simulink model "untitled"  (R2022a)
settings: Solver=VariableStepAuto  StartTime=0.0  StopTime=10  RelTol=1e-3
values from neighbouring files (symbols this model uses):
  C_PM = 1.758e-3    (= 0.001758)    [journal.m]
  Cfilter = 1/(Larm*wc2)    (= 4.78421193241e-05)    [journal.m]
  Cg = 50e-9    (= 5e-08)    [journal.m]
  Fc = Fnom*3.37    (= 168.5)    [journal.m]
  Fnom = 50    [journal.m]
  Inom = Pnom/(sqrt(3)*Vnom_dc)    [journal.m]
  Ki_Ireg = 6    [journal.m]
  Ki_Preg = 1.0    (= 1)    [journal.m]
  Ki_Qreg = 1.0    (= 1)    [journal.m]
  Ki_VDCreg = 100    [journal.m]
  Kp_Ireg = 0.6    [journal.m]
  Kp_Preg = 0.5/3    (= 0.166666666667)    [journal.m]
  Kp_Qreg = 0.5/3    (= 0.166666666667)    [journal.m]
  Kp_VDCreg = 4    [journal.m]
  L_cable = 15e-3    (= 0.015)    [journal.m]
  Larm = Larm_pu*(Zbase/(2*pi*Fnom))    (= 0.0529455974536)    [journal.m]
  Lff = Larm_pu/2    (= 0.075)    [journal.m]
  Lfilter = 0    [journal.m]
  Limits_Ireg = [ 2.0  -2.0]    [journal.m]
  Limits_Preg = [ 1.2, 0.8 ]    [journal.m]
  Limits_Qreg = [ 0.25, -0.25 ]    [journal.m]
  Limits_VDCreg = [ 2.0  -2.0]    [journal.m]
  Lxfo = 0.12    [journal.m]
  Nb_PM = 36    [journal.m]
  Pnom = 1000e6    (= 1000000000)    [journal.m]
  R_cable = 0.5    [journal.m]
  R_startup = 400    [journal.m]
  Rarm = Rarm_pu*Zbase    (= 0.1663335)    [journal.m]
  Rff = Rarm_pu/2    (= 0.00075)    [journal.m]
  Rfilter = 1/(Cfilter*w)*30    (= 1996.002)    [journal.m]
  Rg = 100    [journal.m]
  Rxfo = 0.003    [journal.m]
  Slope_Pref = 0.5    [journal.m]
  Slope_Qref = 0.5    [journal.m]
  Slope_Vdc_ref = Vnom_dc/5    (= 128000)    [journal.m]
  Tbrk1_On = 0.1    [journal.m]
  Tbrk2_On = 0.5    [journal.m]
  Tdeblock = 1    [journal.m]
  Tfault = 999    [journal.m]
  Ton_Converter2 = 2    [journal.m]
  Ton_PQreg = 2    [journal.m]
  Ton_VDCreg = 1    [journal.m]
  Ts = Ts_Control    (= 4e-05)    [journal.m]
  Ts_Control = 40e-6    (= 4e-05)    [journal.m]
  Ts_Power = 20e-6    (= 2e-05)    [journal.m]
  Vnom_dc = 640e3    (= 640000)    [journal.m]
  Vnom_prim = 400e3    (= 400000)    [journal.m]
  Vnom_sec = 333e3    (= 333000)    [journal.m]
undefined symbols (not defined in the file or in its folder): D11, Delta, DiscIntNeverNeededParam, find_system, Pcc, sigbuilder_block
libraries: powerlib_extras x42, spsSeriesRLCBranchLib x32, spsCurrentMeasurementLib x24, simulink x18, spsVoltageMeasurementLib x16, spsHalfBridgeMMCLib x12, spsThreePhaseVIMeasurementLib x10, simulink_extras x6, spsBreakerLib x6, spsParallelRLCBranchLib x6, spsThreePhaseBreakerLib x4, spsMeanLib x4
(part 2 of 6)

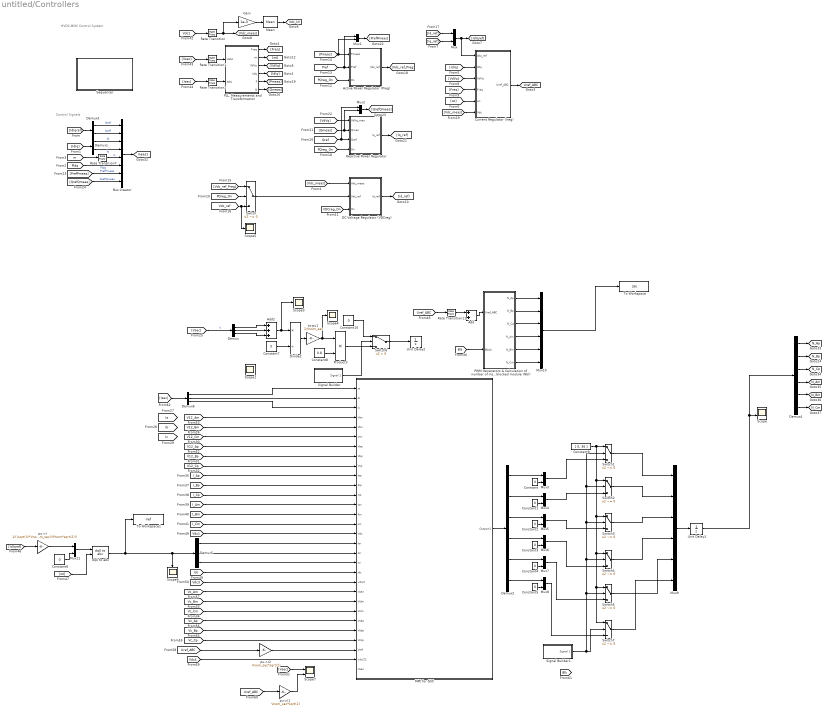
== system untitled/Controllers ==
  note: HVDC-MMC Control System
  note: Control Signals
  Active Power Regulator (Preg) : Subsystem
  Add : Sum
  Add2 : Sum  Inputs=+++
  Bus Creator : BusCreator  Inputs=8
  Constant{,1..6,10} (8 alike) : Constant  Value=0
  Constant7 : Constant  Value=3
  Constant8 : Constant  Value=0.8
  Constant9 : Constant  Value=[ 0, 36 ]
  Current Regulator (Ireg) : Subsystem
  DC Voltage Regulator (VDCreg) : Subsystem
  Demux : Demux  Outputs=3
  Demux1 : Demux  Outputs=2
  Demux2 : Demux  Outputs=6
  Demux3 : Demux  Outputs=2
  Demux4 : Demux  Outputs=6
  Demux5 : Demux  Outputs=3
  Demux6 : Demux  Outputs=3
  Divide2 : Product  Inputs=*/
  Gain : Gain  Gain=1e-3
  MPC for GSC : Subsystem
  Mean : spsMeanLib/Mean  Freq=Fnom/3  Vinit=0  Ts=Ts_Control
  Mux{,1..8,11} (10 alike) : Mux  Inputs=2
  Mux10 : Mux  Inputs=6
  Mux9 : Mux  Inputs=6
  "PLL, Measurements and Transformation" : Subsystem
  PWM Generators & Calculation of number of inserted modules (Nin) and number of blocked module (Nbl) : Subsystem
  Product3 : Product  RndMeth=Zero
  Rate Transition{,1..2,7} (4 alike) : RateTransition  OutPortSampleTime=Ts_Control
  Rate Transition11 : RateTransition  OutPortSampleTime=Ts_Power
  Reactive Power Regulator : Subsystem
  Scope : Scope  NumInputPorts=2
  Scope1 : Scope  NumInputPorts=2
  Scope{3..6} (4 alike) : Scope
  Scope7 : Scope  NumInputPorts=2
  Sequencer : Subsystem
      mask Display: disp('Sequencer')
  Signal Builder : Subsystem  Tag=STV Subsys  LoadFcn=sigbuilder_block('load');  StartFcn=sigbuilder_block('start');  StopFcn=sigbuilder_block('stop');  ClipboardFcn=sigbuilder_block('clipboard');  mask(Sigbuilder block){tuvar=[0:10]}
      mask help: Simulink:masks:SigbuilderBlock_MD
      mask init:
      | if ~strcmp(get_param(bdroot(gcbh),'SimulationStatus'),'stopped') tuvar = sigbuilder_block('maskInit'); end
      settings: CopyFcn=sigbuilder_block('copy');  DeleteFcn=sigbuilder_block('delete');  ModelCloseFcn=sigbuilder_block('modelClose');  PreSaveFcn=sigbuilder_block('preSave');  PauseFcn=sigbuilder_block('pause');  ContinueFcn=sigbuilder_block('continue');  NameChangeFcn=sigbuilder_block('namechange');  OpenFcn=sigbuilder_block('open',[0 36 1152 555.6 ]);  CloseFcn=sigbuilder_block('close');
      mask Display: plot(0, 0, 100, 100,[2, 2, 32, 32, 2], [68, 8, 8, 68, 68],[32, 2], [38, 38], [32, 19, 2],[53, 60, 44], [32, 17, 17, 2],[16, 16, 31, 31]);txt = getActiveGroup(gcbh);text(2, 100, txt,'verticalAlignment', 'top');
  Signal Builder1 : Subsystem  Tag=STV Subsys  LoadFcn=sigbuilder_block('load');  StartFcn=sigbuilder_block('start');  StopFcn=sigbuilder_block('stop');  ClipboardFcn=sigbuilder_block('clipboard');  mask(Sigbuilder block){tuvar=[0:10]}
      mask help: Simulink:masks:SigbuilderBlock_MD
      mask init:
      | if ~strcmp(get_param(bdroot(gcbh),'SimulationStatus'),'stopped') tuvar = sigbuilder_block('maskInit'); end
      settings: CopyFcn=sigbuilder_block('copy');  DeleteFcn=sigbuilder_block('delete');  ModelCloseFcn=sigbuilder_block('modelClose');  PreSaveFcn=sigbuilder_block('preSave');  PauseFcn=sigbuilder_block('pause');  ContinueFcn=sigbuilder_block('continue');  NameChangeFcn=sigbuilder_block('namechange');  OpenFcn=sigbuilder_block('open',[0 36 1152 555.6 ]);  CloseFcn=sigbuilder_block('close');
      mask Display: plot(0, 0, 100, 100,[2, 2, 32, 32, 2], [68, 8, 8, 68, 68],[32, 2], [38, 38], [32, 19, 2],[53, 60, 44], [32, 17, 17, 2],[16, 16, 31, 31]);txt = getActiveGroup(gcbh);text(2, 100, txt,'verticalAlignment', 'top');
  Switch{,1..5,7} (7 alike) : Switch  Criteria=u2 ~= 0  SaturateOnIntegerOverflow=off  InputSameDT=off
  Switch6 : Switch  Criteria=u2 > Threshold  SaturateOnIntegerOverflow=off  InputSameDT=off
  To Workspace : ToWorkspace  VariableName=SM  SaveFormat=Timeseries  SampleTime=-1
  To Workspace1 : ToWorkspace  VariableName=Iref  SaveFormat=Timeseries  SampleTime=-1
  Unit Delay1 : UnitDelay  SampleTime=-1
  Unit Delay2 : UnitDelay  SampleTime=-1
  dq0 to abc : spsdq0toabcLib/dq0 to abc  Alignment=90 degrees behind phase A axis
  pu->I : Gain  Gain=1/((sqrt(3)*Vnom_sec)/(Pnom*sqrt(2)))  SaturateOnIntegerOverflow=on  OutDataTypeStr=Inherit: Same as input  ParamDataTypeStr=Inherit: Same as input
  pu->I1 : Gain  Gain=Vnom_sec*sqrt(2)  SaturateOnIntegerOverflow=on  OutDataTypeStr=Inherit: Same as input  ParamDataTypeStr=Inherit: Same as input
  pu->I2 : Gain  Gain=Vnom_sec*sqrt(2)  SaturateOnIntegerOverflow=on  OutDataTypeStr=Inherit: Same as input  ParamDataTypeStr=Inherit: Same as input
  to-pu1 : Gain  Gain=1/Vnom_sec
  tag scope: N_Am=global, N_Ap=global, N_Bm=global, N_Bp=global, N_Cm=global, N_Cp=global, Uref_ABC=global, Vdc_kV=global, meas1=global
  wires:
  [Uref_ABC] -> Rate Transition11/1
  Mean/1 -> [Vdc_kV]
  [Vsec] -> Rate Transition1/1
  [Isec] -> Rate Transition2/1
  [Vdc_meas] -> Current Regulator (Ireg)/6(Vdc)
  [Vdc_meas] -> DC Voltage Regulator (VDCreg)/1(Vdc_meas)
  DC Voltage Regulator (VDCreg)/1(Id_ref) -> [Id_ref]
  Gain/1 -> Mean/1
  Current Regulator (Ireg)/1(Uref_ABC) -> [Uref_ABC]
  [wt] -> Current Regulator (Ireg)/5(wt)
  [Vdc1] -> Rate Transition/1
  "PLL, Measurements and Transformation"/2(wt) -> [wt]
  "PLL, Measurements and Transformation"/4(IdIq) -> [IdIq]
  [Freq] -> Current Regulator (Ireg)/4(Freq)
  [Id_ref] -> Mux/1
  "PLL, Measurements and Transformation"/3(VdVq) -> [VdVq]
  Mux/1 -> Current Regulator (Ireg)/1(IdIq_ref), [IdIqref]
  Demux1/2 -> Bus Creator/4  "Iq"
  [IdIq] -> Current Regulator (Ireg)/2(IdIq)
  [IdIqref] -> Demux3/1
  Demux3/1 -> Bus Creator/1  "Idref"
  [IdIq] -> Demux1/1
  Bus Creator/1 -> [meas1]
  Demux3/2 -> Bus Creator/2  "Iqref"
  [m] -> Rate Transition7/1
  Demux1/1 -> Bus Creator/3  "Id"
  [PIdq] -> Bus Creator/6  "PIdq"
  "PLL, Measurements and Transformation"/1(Freq) -> [Freq]
  [VdVq] -> Current Regulator (Ireg)/3(VdVq)
  [Iq_ref] -> Mux/2
  Rate Transition/1 -> Gain/1, [Vdc_meas]
  Rate Transition2/1 -> "PLL, Measurements and Transformation"/2(Iabc)
  Rate Transition7/1 -> Bus Creator/5  "m"
  Rate Transition1/1 -> "PLL, Measurements and Transformation"/1(Vabc)
  [Vdc_ref] -> Scope5/1, Switch/3
  [PQreg_On] -> Reactive Power Regulator/4(On)
  Mux2/1 -> [QrefQmeas]
  Mux1/1 -> [PrefPmeas]
  [Vdc_ref_Preg] -> Switch/1
  [Qref] -> Mux2/1, Reactive Power Regulator/3(Qref)
  [QrefQmeas] -> Bus Creator/8  "QrefQmeas"
  [VDCreg_On] -> DC Voltage Regulator (VDCreg)/3(On)
  [PQreg_On] -> Active Power Regulator (Preg)/3(On)
  Active Power Regulator (Preg)/1(Vdc_ref) -> [Vdc_ref_Preg]
  Reactive Power Regulator/1(Iq_ref) -> [Iq_ref]
  "PLL, Measurements and Transformation"/5(P) -> [Pmeas]
  [VdVq] -> Reactive Power Regulator/1(VdVq_mes)
  [Qmeas] -> Mux2/2, Reactive Power Regulator/2(Qmes)
  [PQreg_On] -> Switch/2
  Switch/1 -> DC Voltage Regulator (VDCreg)/2(Vdc_ref)
  [Pref] -> Active Power Regulator (Preg)/2(Pref), Mux1/1
  [PrefPmeas] -> Bus Creator/7  "PrefPmeas"
  "PLL, Measurements and Transformation"/6(Q) -> [Qmeas]
  [Pmeas] -> Active Power Regulator (Preg)/1(Pmeas), Mux1/2
  [Blk] -> PWM Generators & Calculation of number of inserted modules (Nin) and number of blocked module (Nbl)/2(Block)
  Demux/1 -> Add2/1
  Constant10/1 -> Switch6/1
  Constant7/1 -> Divide2/2
  to-pu1/1 -> Scope4/1, Product3/1
  Signal Builder/1(Signal 1) -> Switch6/2
  Demux/2 -> Add2/2
  Demux/3 -> Add2/3
  Add2/1 -> Scope3/1, Divide2/1
  Constant8/1 -> Product3/2
  Switch6/1 -> Unit Delay2/1
  Divide2/1 -> to-pu1/1
  [Vsec] -> Demux/1  "V"
  Rate Transition11/1 -> Add/1
  Add/1 -> PWM Generators & Calculation of number of inserted modules (Nin) and number of blocked module (Nbl)/1(Uref_ABC)
  Product3/1 -> Switch6/3
  PWM Generators & Calculation of number of inserted modules (Nin) and number of blocked module (Nbl)/1(N_Ap) -> Mux10/1
  PWM Generators & Calculation of number of inserted modules (Nin) and number of blocked module (Nbl)/2(N_Bp) -> Mux10/2
  PWM Generators & Calculation of number of inserted modules (Nin) and number of blocked module (Nbl)/3(N_Cp) -> Mux10/3
  PWM Generators & Calculation of number of inserted modules (Nin) and number of blocked module (Nbl)/4(N_Am) -> Mux10/4
  PWM Generators & Calculation of number of inserted modules (Nin) and number of blocked module (Nbl)/5(N_Bm) -> Mux10/5
  PWM Generators & Calculation of number of inserted modules (Nin) and number of blocked module (Nbl)/6(N_Cm) -> Mux10/6
  Demux4/1 -> [N_Ap]
  Demux4/2 -> [N_Bp]
  Demux4/3 -> [N_Cp]
  Demux4/4 -> [N_Am]
  Demux4/5 -> [N_Bm]
  Demux4/6 -> [N_Cm]
  [I_Bm] -> MPC for GSC/14(ibn)
  pu->I/1 -> Mux11/1
  [I_Ap] -> MPC for GSC/10(iap)
  [V12_Bp] -> MPC for GSC/8(Vbp)
  Mux11/1 -> dq0 to abc/1
  Demux2/4 -> Mux6/1
  Demux2/3 -> Mux5/1
  Demux2/5 -> Mux7/1
  Constant/1 -> Mux3/2
  [V12_Cp] -> MPC for GSC/9(Vcp)
  [V12_Bm] -> MPC for GSC/5(Vbn)
  [V12_Ap] -> MPC for GSC/7(Vap)
  Demux2/6 -> Mux8/1
  Constant1/1 -> Mux4/2
  [I_Am] -> MPC for GSC/13(ian)
  [Vdc1] -> MPC for GSC/16(Vdc)
  Demux6/2 -> MPC for GSC/2(ib)
  Demux5/2 -> MPC for GSC/18(ibr)
  Demux5/1 -> MPC for GSC/17(iar)
  Constant5/1 -> Mux8/2
  [wt] -> dq0 to abc/2
  Demux6/3 -> MPC for GSC/3(ic)
  Demux2/2 -> Mux4/1
  Constant4/1 -> Mux7/2
  [I_Bp] -> MPC for GSC/11(ibp)
  [IdIqref] -> pu->I/1
  [V12_Cm] -> MPC for GSC/6(Vcn)
  Constant6/1 -> Mux11/2
  Constant3/1 -> Mux6/2
  Demux5/3 -> MPC for GSC/19(icr)
  [V12_Am] -> MPC for GSC/4(Van)
  MPC for GSC/1(Outport1) -> Demux2/1
  Demux6/1 -> MPC for GSC/1(ia)
  [I_Cp] -> MPC for GSC/12(icp)
  [I_Cm] -> MPC for GSC/15(icn)
  Mux9/1 -> Unit Delay1/1
  Constant2/1 -> Mux5/2
  [Idc] -> MPC for GSC/20(idc)
  [Vdc3] -> MPC for GSC/21(vdc/2)
  [Vc_Am] -> MPC for GSC/22(Vcan)
  [Vc_Bm] -> MPC for GSC/23(Vcbn)
  [Vc_Cm] -> MPC for GSC/24(Vccn)
  [Vc_Ap] -> MPC for GSC/25(Vcap)
  [Vc_Bp] -> MPC for GSC/26(Vcbp)
  [Vc_Cp] -> MPC for GSC/27(Vccp)
  [Vdc4] -> MPC for GSC/29(vdc/21)
  [Uref_ABC] -> pu->I1/1
  Demux2/1 -> Mux3/1
  Mux10/1 -> To Workspace/1
  Mux7/1 -> Switch5/3
  Mux4/1 -> Switch2/3
  Mux6/1 -> Switch4/3
  Signal Builder1/1(Signal 1) -> Switch1/2, Switch2/2, Switch3/2, Switch4/2, Switch5/2, Switch7/2
  Mux8/1 -> Switch7/3
  Switch7/1 -> Mux9/6
  Switch4/1 -> Mux9/4
  Switch5/1 -> Mux9/5
  Mux3/1 -> Switch1/3
  Switch2/1 -> Mux9/2
  Mux5/1 -> Switch3/3
  Constant9/1 -> Switch1/1, Switch7/1, Switch5/1, Switch4/1, Switch3/1, Switch2/1
  Switch3/1 -> Mux9/3
  Switch1/1 -> Mux9/1
  pu->I1/1 -> Scope7/2
  ? -> MPC for GSC/30(Vsec)
  [Vsec] -> Scope7/1
  [Uref_ABC] -> pu->I2/1
  pu->I2/1 -> MPC for GSC/28(Vref)
  [Isec] -> Demux6/1
  Unit Delay1/1 -> Demux4/1, Scope/2
  ? -> Scope/1
  dq0 to abc/1 -> To Workspace1/1, Demux5/1, Scope6/1

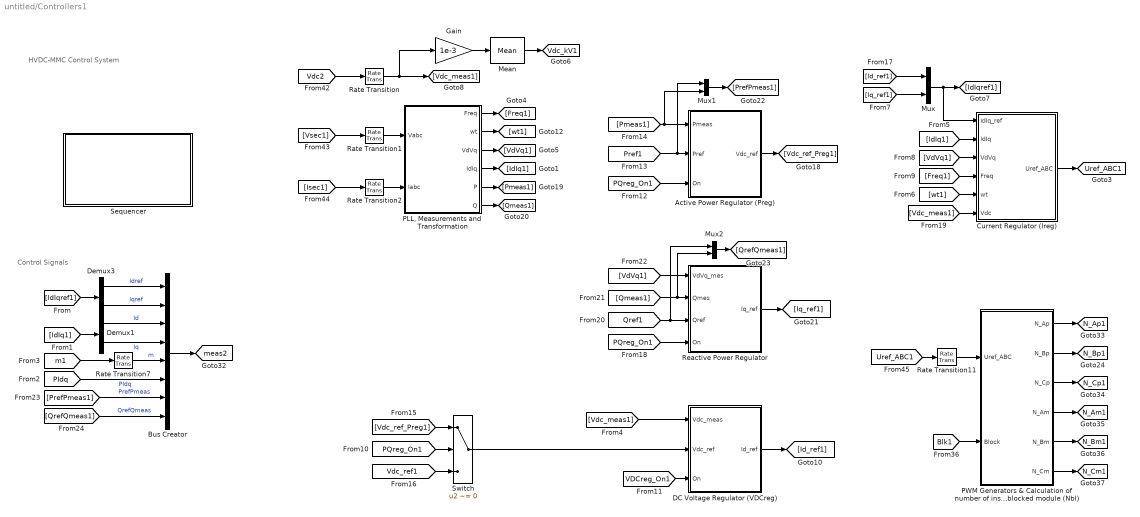
== system untitled/Controllers1 ==
  note: HVDC-MMC Control System
  note: Control Signals
  Active Power Regulator (Preg) : Subsystem
  Bus Creator : BusCreator  Inputs=8
  Current Regulator (Ireg) : Subsystem
  DC Voltage Regulator (VDCreg) : Subsystem
  Demux1 : Demux  Outputs=2
  Demux3 : Demux  Outputs=2
  Gain : Gain  Gain=1e-3
  Mean : spsMeanLib/Mean  Freq=Fnom/3  Vinit=0  Ts=Ts_Control
  Mux : Mux  Inputs=2
  Mux1 : Mux  Inputs=2
  Mux2 : Mux  Inputs=2
  "PLL, Measurements and Transformation" : Subsystem
  PWM Generators & Calculation of number of inserted modules (Nin) and number of blocked module (Nbl) : Subsystem
  Rate Transition{,1..2,7} (4 alike) : RateTransition  OutPortSampleTime=Ts_Control
  Rate Transition11 : RateTransition  OutPortSampleTime=Ts_Power
  Reactive Power Regulator : Subsystem
  Sequencer : Subsystem
      mask Display: disp('Sequencer')
  Switch : Switch  Criteria=u2 ~= 0  SaturateOnIntegerOverflow=off  InputSameDT=off
  tag scope: N_Am1=global, N_Ap1=global, N_Bm1=global, N_Bp1=global, N_Cm1=global, N_Cp1=global, Uref_ABC1=global, Vdc_kV1=global, meas2=global
  wires:
  Rate Transition11/1 -> PWM Generators & Calculation of number of inserted modules (Nin) and number of blocked module (Nbl)/1(Uref_ABC)
  [Uref_ABC1] -> Rate Transition11/1
  Mean/1 -> [Vdc_kV1]
  [Vsec1] -> Rate Transition1/1
  [Isec1] -> Rate Transition2/1
  [Vdc_meas1] -> Current Regulator (Ireg)/6(Vdc)
  [Vdc_meas1] -> DC Voltage Regulator (VDCreg)/1(Vdc_meas)
  DC Voltage Regulator (VDCreg)/1(Id_ref) -> [Id_ref1]
  Gain/1 -> Mean/1
  Current Regulator (Ireg)/1(Uref_ABC) -> [Uref_ABC1]
  [wt1] -> Current Regulator (Ireg)/5(wt)
  [Vdc2] -> Rate Transition/1
  "PLL, Measurements and Transformation"/2(wt) -> [wt1]
  "PLL, Measurements and Transformation"/4(IdIq) -> [IdIq1]
  [Freq1] -> Current Regulator (Ireg)/4(Freq)
  [Id_ref1] -> Mux/1
  "PLL, Measurements and Transformation"/3(VdVq) -> [VdVq1]
  Mux/1 -> Current Regulator (Ireg)/1(IdIq_ref), [IdIqref1]
  Demux1/2 -> Bus Creator/4  "Iq"
  [IdIq1] -> Current Regulator (Ireg)/2(IdIq)
  [IdIqref1] -> Demux3/1
  Demux3/1 -> Bus Creator/1  "Idref"
  [IdIq1] -> Demux1/1
  Bus Creator/1 -> [meas2]
  Demux3/2 -> Bus Creator/2  "Iqref"
  [m1] -> Rate Transition7/1
  Demux1/1 -> Bus Creator/3  "Id"
  [PIdq] -> Bus Creator/6  "PIdq"
  "PLL, Measurements and Transformation"/1(Freq) -> [Freq1]
  [VdVq1] -> Current Regulator (Ireg)/3(VdVq)
  [Iq_ref1] -> Mux/2
  Rate Transition/1 -> Gain/1, [Vdc_meas1]
  Rate Transition2/1 -> "PLL, Measurements and Transformation"/2(Iabc)
  Rate Transition7/1 -> Bus Creator/5  "m"
  Rate Transition1/1 -> "PLL, Measurements and Transformation"/1(Vabc)
  [Vdc_ref1] -> Switch/3
  [PQreg_On1] -> Reactive Power Regulator/4(On)
  Mux2/1 -> [QrefQmeas1]
  Mux1/1 -> [PrefPmeas1]
  [Vdc_ref_Preg1] -> Switch/1
  [Qref1] -> Mux2/1, Reactive Power Regulator/3(Qref)
  [QrefQmeas1] -> Bus Creator/8  "QrefQmeas"
  [VDCreg_On1] -> DC Voltage Regulator (VDCreg)/3(On)
  [PQreg_On1] -> Active Power Regulator (Preg)/3(On)
  Active Power Regulator (Preg)/1(Vdc_ref) -> [Vdc_ref_Preg1]
  Reactive Power Regulator/1(Iq_ref) -> [Iq_ref1]
  "PLL, Measurements and Transformation"/5(P) -> [Pmeas1]
  [VdVq1] -> Reactive Power Regulator/1(VdVq_mes)
  [Qmeas1] -> Mux2/2, Reactive Power Regulator/2(Qmes)
  [PQreg_On1] -> Switch/2
  Switch/1 -> DC Voltage Regulator (VDCreg)/2(Vdc_ref)
  [Pref1] -> Active Power Regulator (Preg)/2(Pref), Mux1/1
  [PrefPmeas1] -> Bus Creator/7  "PrefPmeas"
  "PLL, Measurements and Transformation"/6(Q) -> [Qmeas1]
  [Pmeas1] -> Active Power Regulator (Preg)/1(Pmeas), Mux1/2
  PWM Generators & Calculation of number of inserted modules (Nin) and number of blocked module (Nbl)/1(N_Ap) -> [N_Ap1]
  PWM Generators & Calculation of number of inserted modules (Nin) and number of blocked module (Nbl)/2(N_Bp) -> [N_Bp1]
  PWM Generators & Calculation of number of inserted modules (Nin) and number of blocked module (Nbl)/3(N_Cp) -> [N_Cp1]
  PWM Generators & Calculation of number of inserted modules (Nin) and number of blocked module (Nbl)/4(N_Am) -> [N_Am1]
  PWM Generators & Calculation of number of inserted modules (Nin) and number of blocked module (Nbl)/5(N_Bm) -> [N_Bm1]
  PWM Generators & Calculation of number of inserted modules (Nin) and number of blocked module (Nbl)/6(N_Cm) -> [N_Cm1]
  [Blk1] -> PWM Generators & Calculation of number of inserted modules (Nin) and number of blocked module (Nbl)/2(Block)

== system untitled/DC & converter 1 ==
  CnDC : spsSeriesRLCBranchLib/Series RLC Branch  LConnTagsString=__new0  RConnTagsString=__new0  BranchType=RC  Resistance=Rg  Inductance=1e-3  SetiL0=off  InitialCurrent=0  Capacitance=Cg  Setx0=off  InitialVoltage=Vnom_dc/2  Measurements=None
  CpDC : spsSeriesRLCBranchLib/Series RLC Branch  LConnTagsString=__new0  RConnTagsString=__new0  BranchType=RC  Resistance=Rg  Inductance=1e-3  SetiL0=off  InitialCurrent=0  Capacitance=Cg  Setx0=off  InitialVoltage=Vnom_dc/2  Measurements=None
  Current Measurement2 : spsCurrentMeasurementLib/Current Measurement  PhasorSimulation=off  OutputType=Complex  PSBequivalent=0
  Gain2 : Gain  Gain=1e-3
  Gain3 : Gain  Gain=1e-3
  Ground4 : spsGroundLib/Ground  LConnTagsString=a
  Idc (kA)1 : Display
      settings: Format=bank  Decimation=5000
  P (MW)1 : Display
      settings: Format=bank  Decimation=5000
  Product1 : Product
  Vdc (kV)1 : Display
      settings: Format=bank  Decimation=5000
  Voltage Measurement2 : spsVoltageMeasurementLib/Voltage Measurement  PhasorSimulation=off  OutputType=Complex  PSBequivalent=0
  1 : PMIOPort  Side=Left
  2 : PMIOPort  Port=2  Side=Left
  5 : PMIOPort  Port=3  Side=Right
  6 : PMIOPort  Port=4  Side=Right
  tag scope: Idc2=global, Vdc2=global
  wires:
  Voltage Measurement2/1 -> [Vdc2]
  Current Measurement2/1 -> [Idc2]
  Gain2/1 -> Product1/1, Vdc (kV)1/1
  Product1/1 -> P (MW)1/1
  [Vdc2] -> Gain2/1
  [Idc2] -> Gain3/1
  Gain3/1 -> Product1/2, Idc (kA)1/1
  connections:
  Ground4/LConn1 -- CnDC/LConn1 -- CpDC/RConn1
  CnDC/RConn1 -- 6/RConn1 -- Voltage Measurement2/LConn2 -- 2/RConn1
  Voltage Measurement2/LConn1 -- Current Measurement2/RConn1 -- 5/RConn1 -- CpDC/LConn1
  1/RConn1 -- Current Measurement2/LConn1

== system untitled/DC & converter 2 ==
  note: Cable (simplified model)
  On : Inport
  Fault : Inport  Port=2
  CnDC : spsSeriesRLCBranchLib/Series RLC Branch  LConnTagsString=__new0  RConnTagsString=__new0  BranchType=RC  Resistance=Rg  Inductance=1e-3  SetiL0=off  InitialCurrent=0  Capacitance=Cg  Setx0=off  InitialVoltage=Vnom_dc/2  Measurements=None
  CpDC : spsSeriesRLCBranchLib/Series RLC Branch  LConnTagsString=__new0  RConnTagsString=__new0  BranchType=RC  Resistance=Rg  Inductance=1e-3  SetiL0=off  InitialCurrent=0  Capacitance=Cg  Setx0=off  InitialVoltage=Vnom_dc/2  Measurements=None
  Current Measurement2 : spsCurrentMeasurementLib/Current Measurement  PhasorSimulation=off  OutputType=Complex  PSBequivalent=0
  Gain2 : Gain  Gain=1e-3
  Gain3 : Gain  Gain=1e-3
  Ground2 : spsGroundLib/Ground  LConnTagsString=a
  Ground4 : spsGroundLib/Ground  LConnTagsString=a
  Idc (kA)1 : Display
      settings: Format=bank  Decimation=5000
  Ideal Switch : spsIdealSwitchLib/Ideal Switch  Ron=0.001  Lon=0  IC=0  Rs=1e6  Cs=inf  Measurements=off
  Ideal Switch1 : spsIdealSwitchLib/Ideal Switch  Ron=0.001  Lon=0  IC=0  Rs=1e6  Cs=inf  Measurements=off
  P (MW)1 : Display
      settings: Format=bank  Decimation=5000
  Product1 : Product
  Sw_Fault : spsIdealSwitchLib/Ideal Switch  Ron=Rfault  Lon=0  IC=0  Rs=1e6  Cs=inf  Measurements=off
  Vdc (kV)1 : Display
      settings: Format=bank  Decimation=5000
  Voltage Measurement1 : spsVoltageMeasurementLib/Voltage Measurement  PhasorSimulation=off  OutputType=Complex  PSBequivalent=0
  Voltage Measurement2 : spsVoltageMeasurementLib/Voltage Measurement  PhasorSimulation=off  OutputType=Complex  PSBequivalent=0
  Voltage Measurement3 : spsVoltageMeasurementLib/Voltage Measurement  PhasorSimulation=off  OutputType=Complex  PSBequivalent=0
  Zcable1_1 : spsSeriesRLCBranchLib/Series RLC Branch  LConnTagsString=__new0  RConnTagsString=__new0  BranchType=RL  Resistance=R_cable/2  Inductance=L_cable/2  SetiL0=off  InitialCurrent=0  Capacitance=1e-6  Setx0=off  InitialVoltage=0  Measurements=None
  Zcable1_2 : spsSeriesRLCBranchLib/Series RLC Branch  LConnTagsString=__new0  RConnTagsString=__new0  BranchType=RL  Resistance=R_cable/2  Inductance=L_cable/2  SetiL0=off  InitialCurrent=0  Capacitance=1e-6  Setx0=off  InitialVoltage=0  Measurements=None
  Zcable2_1 : spsSeriesRLCBranchLib/Series RLC Branch  LConnTagsString=__new0  RConnTagsString=__new0  BranchType=RL  Resistance=R_cable/2  Inductance=L_cable/2  SetiL0=off  InitialCurrent=0  Capacitance=1e-6  Setx0=off  InitialVoltage=0  Measurements=None
  Zcable2_2 : spsSeriesRLCBranchLib/Series RLC Branch  LConnTagsString=__new0  RConnTagsString=__new0  BranchType=RL  Resistance=R_cable/2  Inductance=L_cable/2  SetiL0=off  InitialCurrent=0  Capacitance=1e-6  Setx0=off  InitialVoltage=0  Measurements=None
  1 : PMIOPort  Side=Left
  2 : PMIOPort  Port=2  Side=Left
  5 : PMIOPort  Port=3  Side=Right
  6 : PMIOPort  Port=4  Side=Right
  tag scope: Idc1=global, Vdc1=global, Vdc3=global, Vdc4=global
  wires:
  Gain2/1 -> Product1/1, Vdc (kV)1/1
  Product1/1 -> P (MW)1/1
  [Vdc1] -> Gain2/1
  [Idc1] -> Gain3/1
  Gain3/1 -> Product1/2, Idc (kA)1/1
  On/1 -> Ideal Switch1/1, Ideal Switch/1
  Fault/1 -> Sw_Fault/1
  Voltage Measurement2/1 -> [Vdc1]
  Current Measurement2/1 -> [Idc1]
  Voltage Measurement1/1 -> [Vdc3]
  Voltage Measurement3/1 -> [Vdc4]
  connections:
  Ground4/LConn1 -- CnDC/LConn1 -- CpDC/RConn1
  Zcable2_1/RConn1 -- 2/RConn1 -- CnDC/RConn1
  Zcable2_2/RConn1 -- Sw_Fault/RConn1 -- Voltage Measurement3/LConn2 -- Voltage Measurement2/LConn2 -- Zcable2_1/LConn1
  Zcable1_1/RConn1 -- CpDC/LConn1 -- 1/RConn1
  Voltage Measurement2/LConn1 -- Current Measurement2/RConn1 -- Voltage Measurement1/LConn1 -- Zcable1_2/RConn1 -- Sw_Fault/LConn1
  Ideal Switch/LConn1 -- Zcable1_2/LConn1
  Ideal Switch1/LConn1 -- Zcable2_2/LConn1
  5/RConn1 -- Ideal Switch/RConn1
  Ideal Switch1/RConn1 -- 6/RConn1
  Current Measurement2/LConn1 -- Zcable1_1/LConn1
  Ground2/LConn1 -- Voltage Measurement3/LConn1 -- Voltage Measurement1/LConn2

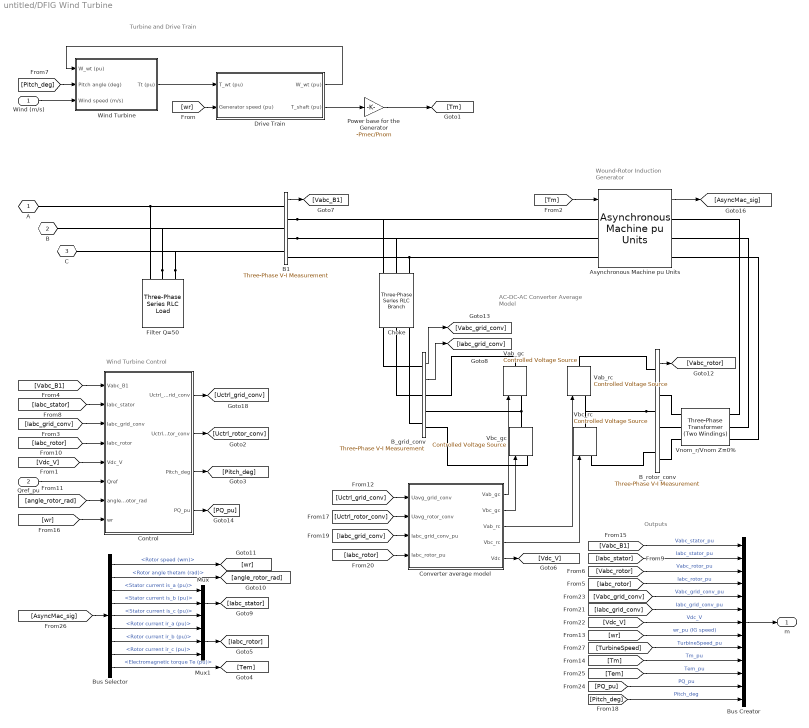
== system untitled/DFIG Wind Turbine ==
  note: Turbine and Drive Train
  note: Wind Turbine Control
  note: Wound-Rotor
      | Induction Generator
  note: AC-DC-AC Converter
      | Average Model
  note: Outputs
  "Wind (m/s) " : Inport
  Qref_pu : Inport  Port=2
  Asynchronous Machine pu Units : spsAsynchronousMachinepuUnitsLib/Asynchronous Machine pu Units  RotorType=Wound  PresetModel=No  MechanicalLoad=Torque Tm  ShowDetailedParameters=on  ReferenceFrame=Rotor  Units=pu  MeasurementBus=off  NominalParameters=[ Pnom Vnom Fnom ]  VoltageRatio=1  Stator=[ Rs Lls]  Rotor=[ Rr Llr]  Cage1=[0.01909 0.0397]  Cage2=[0.01909 0.0397]  Lm=Lm  Mechanical=[H F p]  PolePairs=3  InitialConditions=init  SimulateSaturation=off  Saturation="[0.212,0.4201,0.8125,1.0979,1.4799,2.2457,3.2586,4.5763,6.4763 ;   0.5,0.7,0.9,1,1.1,1.2 ,1.3,1.4,1.5]"  LoadFlowParameters=0  TsPowergui=0  TsBlock=-1  IterativeModel=Trapezoidal non iterative  IterativeDiscreteModel=Trapezoidal non iterative  Pmec=0
      settings: SourceProductBaseCode=PS
  B1 : spsThreePhaseVIMeasurementLib/Three-Phase V-I Measurement  VoltageMeasurement=phase-to-ground  SetLabelV=off  LabelV=Vabc  Vpu=on  VpuLL=off  CurrentMeasurement=no  SetLabelI=on  LabelI=Iabc_B1  Ipu=on  Pbase=Pnom  Vbase=Vnom  OutputType=Complex  PhasorSimulation=off  PSBequivalent=0
  B_grid_conv : spsThreePhaseVIMeasurementLib/Three-Phase V-I Measurement  VoltageMeasurement=phase-to-ground  SetLabelV=off  LabelV=Vabc_B1  Vpu=on  VpuLL=off  CurrentMeasurement=yes  SetLabelI=off  LabelI=Iabc  Ipu=on  Pbase=Pnom  Vbase=Vnom  OutputType=Complex  PhasorSimulation=off  PSBequivalent=0
  B_rotor_conv : spsThreePhaseVIMeasurementLib/Three-Phase V-I Measurement  VoltageMeasurement=phase-to-phase  SetLabelV=off  LabelV=Vabc_B1  Vpu=on  VpuLL=off  CurrentMeasurement=no  SetLabelI=off  LabelI=Iabc  Ipu=on  Pbase=Pnom  Vbase=Vnom_r  OutputType=Complex  PhasorSimulation=off  PSBequivalent=0
  Bus Creator : BusCreator  Inputs=13
  Bus Selector : BusSelector  OutputSignals=Mechanical.Rotor speed (wm),Mechanical.Rotor angle thetam (rad),Stator measurements.Stator current is_a (pu),Stator measurements.Stator current is_b (pu),Stator measurements.Stator current is_c (pu),Rotor measurements.Rotor current ir_a (pu),Rotor measurements.Rotor current ir_b (pu),Rotor measurements.Rotor current ir_c (pu),Mechanical.Electromagnetic torque Te (pu)
  "Choke " : spsThreePhaseSeriesRLCBranchLib/Three-Phase Series RLC Branch  LConnTagsString=A|B|C  RConnTagsString=A|B|C  BranchType=RL  Resistance=R_RL*Vnom^2/Pnom  Inductance=L_RL*Vnom^2/Pnom/(2*pi*Fnom)  Capacitance=[]  Measurements=None
  Control : Subsystem
  Converter average model : Subsystem
  Drive Train : Subsystem  mask(Wind Turbine shaft){H_WT=H_WT, Ksh=Ksh, D_mutual=D_mutual, wbase=2*pi*Fnom/p, w_wt0=w_wt0, torque0=torque0, Ts=Ts}
      mask prompts: H_WT "Wind turbine inertia constant H (s):"; Ksh "Shaft spring constant (pu of nominal mechanical torque/rad):"; D_mutual "Shaft mutual damping (pu of nominal mechanical torque/pu dw):"; wbase "Shaft base speed (rad/s):"; w_wt0 "Turbine initial speed (pu of base speed):"; torque0 "Initial output torque (pu of nominal mechanical torque):"; Ts "Sample time (s):"
      mask help:
      | This block implements a wind turbine drive train model. All shaft parameters are referred to high-speed shaft (generator shaft).
      |
      | The first input is the wind turbine torque in per unit (pu) based on the nominal power of the turbine and the base speed of the generator. The second input is the generator speed in pu based on the base speed of the generator.
      |
      | The outputs are:
      | 1- the transmitted torque of the shaft in pu based on the nominal power of the turbine and the base speed of the generator.
      | 2- the wind turbine speed in pu of the base speed of the generator.
  Filter Q=50 : spsThreePhaseSeriesRLCLoadLib/Three-Phase Series RLC Load  LConnTagsString=A|B|C  Configuration=Y (grounded)  NominalVoltage=Vnom  Vabc=[1e3 1e3 1e3]  Vabcp=[1e3 1e3 1e3]  NominalFrequency=Fnom  UnbalancedPower=off  ActivePower=C_var_filter/Q_filter  InductivePower=0  CapacitivePower=C_var_filter  Pabc=[10e3 9e3 11e3]  QLabc=[100 90 110]  QCabc=[100 90 110]  Pabcp=[10e3 9e3 11e3]  QLabcp=[100 90 110]  QCabcp=[100 90 110]  Measurements=None  LoadType=constant Z
  Mux : Mux  Inputs=3
  Mux1 : Mux  Inputs=3
  Power base for the Generator : Gain  Gain=-Pmec/Pnom  SaturateOnIntegerOverflow=on  OutDataTypeStr=Inherit: Same as input  ParamDataTypeStr=Inherit: Same as input
  Vab_gc : spsControlledVoltageSourceLib/Controlled Voltage Source  Initialize=on  Source_Type=AC  Amplitude=0  Phase=0  Frequency=0  Measurements=None
  Vab_rc : spsControlledVoltageSourceLib/Controlled Voltage Source  Initialize=on  Source_Type=AC  Amplitude=0  Phase=0  Frequency=0  Measurements=None
  Vbc_gc : spsControlledVoltageSourceLib/Controlled Voltage Source  Initialize=on  Source_Type=AC  Amplitude=0  Phase=0  Frequency=0  Measurements=None
  Vbc_rc : spsControlledVoltageSourceLib/Controlled Voltage Source  Initialize=on  Source_Type=AC  Amplitude=0  Phase=0  Frequency=0  Measurements=None
  Vnom_r/Vnom Z=0% : spsThreePhaseTransformerTwoWindingsLib/Three-Phase Transformer (Two Windings)  Winding1Connection=Y  Winding2Connection=Y  CoreType=Three single-phase transformers  SetSaturation=off  Hysteresis=off  DataFile='hysteresis'  SetInitialFlux=off  Measurements=None  UNITS=pu  NominalPower=[ Pnom , Fnom ]  Winding1=[ Vnom_r , 0, 0]  Winding2=[ Vnom , 0, 0]  Rm=500  Lm=inf  L0=0.5  Saturation=[ 0,0 ; 0.0024,1.2 ; 1.0,1.52 ]  InitialFluxes=[ 0.8 , -0.8 , 0.7 ]  BreakLoop=off  DiscreteSolver=Trapezoidal iterative  DataType=off  TransfoNumber=0
  Wind Turbine : Subsystem  mask(Wind Turbine){Prated=Pmec, c1_c8=c1_c8, K1_K2=K1_K2, wind0=wind0, Ts=Ts}
      mask prompts: Prated "Nominal mechanical output power (W):"; c1_c8 "Coefficients [c1 ... c8]"; K1_K2 "Parameters [K1 K2]"; wind0 "Initial wind speed (m/s):"; Ts "Sample time (s):"
      mask help:
      | This block implements a generic wind turbine models.
      |
      | The first input is the turbine speed in per unit of the generator base speed. For a synchronous or asynchronous generator, the base speed is the synchronous speed. For a permanent-magnet generator, the base speed is defined as the speed producing nominal voltage at  no load. The second input is the blade pitch angle in degrees. The third input is the wind speed in m/s.
      |
      | The output is the torque applied to the drive train in per unit based on the nominal power of the turbine and the base speed of the generator.
      mask init:
      | c1 = c1_c8(1);
      | c2 = c1_c8(2);
      | c3 = c1_c8(3);
      | c4 = c1_c8(4);
      | c5 = c1_c8(5);
      | c6 = c1_c8(6);
      | c7 = c1_c8(7);;
      | c8 = c1_c8(8);
      | 
      | K1=K1_K2(1);
      | K2=K1_K2(2);
      settings: OpenFcn=power_openblockproxy();
      mask Display: disp('');
  A : PMIOPort  Tag=PMCPort  Side=Left
  B : PMIOPort  Tag=PMCPort  Port=2  Side=Left
  C : PMIOPort  Tag=PMCPort  Port=3  Side=Left
  m : Outport  VectorParamsAs1DForOutWhenUnconnected=off
  wires:
  [Pitch_deg] -> Bus Creator/13  "Pitch_deg"
  [PQ_pu] -> Bus Creator/12  "PQ_pu"
  Control/4(PQ_pu) -> [PQ_pu]
  [Tem] -> Bus Creator/11  "Tem_pu"
  [Tm] -> Bus Creator/10  "Tm_pu"
  [TurbineSpeed] -> Bus Creator/9  "TurbineSpeed_pu"
  [Vdc_V] -> Bus Creator/7  "Vdc_V"
  [Iabc_grid_conv] -> Bus Creator/6  "Iabc_grid_conv_pu"
  [Vabc_grid_conv] -> Bus Creator/5  "Vabc_grid_conv_pu"
  [Iabc_rotor] -> Bus Creator/4  "Iabc_rotor_pu"
  [Vabc_rotor] -> Bus Creator/3  "Vabc_rotor_pu"
  [Iabc_stator] -> Bus Creator/2  "Iabc_stator_pu"
  [Vabc_B1] -> Bus Creator/1  "Vabc_stator_pu"
  Asynchronous Machine pu Units/1 -> [AsyncMac_sig]
  Converter average model/5(Vdc) -> [Vdc_V]
  Converter average model/4(Vbc_rc) -> Vbc_rc/1
  Converter average model/3(Vab_rc) -> Vab_rc/1
  Converter average model/2(Vbc_gc) -> Vbc_gc/1
  Converter average model/1(Vab_gc) -> Vab_gc/1
  [Uctrl_rotor_conv] -> Converter average model/2(Uavg_rotor_conv)
  [Uctrl_grid_conv] -> Converter average model/1(Uavg_grid_conv)
  [Iabc_rotor] -> Converter average model/4(Iabc_rotor_pu)
  [Iabc_grid_conv] -> Converter average model/3(Iabc_grid_conv_pu)
  [Pitch_deg] -> Wind Turbine/2(Pitch angle (deg))
  Drive Train/1(W_wt (pu)) -> Wind Turbine/1(W_wt (pu))
  "Wind (m/s) "/1 -> Wind Turbine/3(Wind speed (m/s))
  Power base for the Generator/1 -> [Tm]
  Drive Train/2(T_shaft (pu)) -> Power base for the Generator/1
  [wr] -> Drive Train/2(Generator speed (pu))
  Wind Turbine/1(Tt (pu)) -> Drive Train/1(T_wt (pu))
  Qref_pu/1 -> Control/6(Qref)
  Bus Selector/9 -> [Tem]  "<Electromagnetic torque Te (pu)>"
  Bus Selector/1 -> [wr]  "<Rotor speed (wm)>"
  Bus Creator/1 -> m/1
  B_rotor_conv/1 -> [Vabc_rotor]
  B1/1 -> [Vabc_B1]
  [Vabc_B1] -> Control/1(Vabc_B1)
  [Iabc_grid_conv] -> Control/3(Iabc_grid_conv)
  [Iabc_rotor] -> Control/4(Iabc_rotor)
  [angle_rotor_rad] -> Control/7(angle_rotor_rad)
  Mux1/1 -> [Iabc_rotor]
  Mux/1 -> [Iabc_stator]
  [Vdc_V] -> Control/5(Vdc_V)
  Control/3(Pitch_deg) -> [Pitch_deg]
  [Iabc_stator] -> Control/2(Iabc_stator)
  [wr] -> Control/8(wr)
  Bus Selector/8 -> Mux1/3  "<Rotor current ir_c (pu)>"
  Bus Selector/7 -> Mux1/2  "<Rotor current ir_b (pu)>"
  Bus Selector/6 -> Mux1/1  "<Rotor current ir_a (pu)>"
  Bus Selector/5 -> Mux/3  "<Stator current is_c (pu)>"
  Bus Selector/4 -> Mux/2  "<Stator current is_b (pu)>"
  Bus Selector/3 -> Mux/1  "<Stator current is_a (pu)>"
  Bus Selector/2 -> [angle_rotor_rad]  "<Rotor angle thetam (rad)>"
  B_grid_conv/2 -> [Iabc_grid_conv]
  B_grid_conv/1 -> [Vabc_grid_conv]
  Control/1(Uctrl_grid_conv) -> [Uctrl_grid_conv]
  Control/2(Uctrl_rotor_conv) -> [Uctrl_rotor_conv]
  [AsyncMac_sig] -> Bus Selector/1
  [wr] -> Bus Creator/8  "wr_pu (IG speed)"
  [Tm] -> Asynchronous Machine pu Units/1
  connections:
  Filter Q=50/LConn3 -- B1/LConn3 -- C/RConn1
  Filter Q=50/LConn2 -- B1/LConn2 -- B/RConn1
  Filter Q=50/LConn1 -- B1/LConn1 -- A/RConn1
  Vbc_rc/LConn1 -- B_rotor_conv/LConn3
  Vab_rc/RConn1 -- B_rotor_conv/LConn1
  B_rotor_conv/LConn2 -- Vab_rc/LConn1 -- Vbc_rc/RConn1
  B_grid_conv/RConn3 -- Vbc_gc/LConn1
  Vab_gc/RConn1 -- B_grid_conv/RConn1
  B_grid_conv/RConn2 -- Vbc_gc/RConn1 -- Vab_gc/LConn1
  B_rotor_conv/RConn3 -- Vnom_r/Vnom Z=0%/LConn3
  B_rotor_conv/RConn2 -- Vnom_r/Vnom Z=0%/LConn2
  B_rotor_conv/RConn1 -- Vnom_r/Vnom Z=0%/LConn1
  B1/RConn3 -- "Choke "/LConn3 -- Asynchronous Machine pu Units/LConn3
  B1/RConn1 -- "Choke "/LConn1 -- Asynchronous Machine pu Units/LConn1
  Asynchronous Machine pu Units/RConn3 -- Vnom_r/Vnom Z=0%/RConn3
  Asynchronous Machine pu Units/RConn1 -- Vnom_r/Vnom Z=0%/RConn1
  Asynchronous Machine pu Units/RConn2 -- Vnom_r/Vnom Z=0%/RConn2
  "Choke "/RConn3 -- B_grid_conv/LConn3
  "Choke "/RConn2 -- B_grid_conv/LConn2
  "Choke "/RConn1 -- B_grid_conv/LConn1
  B1/RConn2 -- "Choke "/LConn2 -- Asynchronous Machine pu Units/LConn2

== system untitled/Filter ==
  Breaker : spsBreakerLib/Breaker  InitialState=1  SwitchingTimes=Topen_Filter  External=off  BreakerResistance=0.001  SnubberResistance=1e6  SnubberCapacitance=inf  Measurements=None  MoreParameters=on  NoBreakLoop=off
      settings: SourceProductBaseCode=PS
  Current Measurement6 : spsCurrentMeasurementLib/Current Measurement  PhasorSimulation=off  OutputType=Complex  PSBequivalent=0
  Parallel RLC Branch : spsParallelRLCBranchLib/Parallel RLC Branch  LConnTagsString=a  RConnTagsString=__new0  BranchType=RC  Resistance=Rfilter  Inductance=1e-3  SetiL0=off  InitialCurrent=0  Capacitance=Cfilter  Setx0=off  InitialVoltage=0  Measurements=None
  1 : PMIOPort  Side=Left
  2 : PMIOPort  Port=2  Side=Left
  tag scope: Ifilter_A=global
  wires:
  Current Measurement6/1 -> [Ifilter_A]
  connections:
  Parallel RLC Branch/RConn1 -- 2/RConn1
  Current Measurement6/RConn1 -- Parallel RLC Branch/LConn1
  1/RConn1 -- Breaker/LConn1
  Breaker/RConn1 -- Current Measurement6/LConn1

== system untitled/Filter1 ==
  Breaker : spsBreakerLib/Breaker  InitialState=1  SwitchingTimes=Topen_Filter  External=off  BreakerResistance=0.001  SnubberResistance=1e6  SnubberCapacitance=inf  Measurements=None  MoreParameters=on  NoBreakLoop=off
      settings: SourceProductBaseCode=PS
  Current Measurement6 : spsCurrentMeasurementLib/Current Measurement  PhasorSimulation=off  OutputType=Complex  PSBequivalent=0
  Parallel RLC Branch : spsParallelRLCBranchLib/Parallel RLC Branch  LConnTagsString=a  RConnTagsString=__new0  BranchType=RC  Resistance=Rfilter  Inductance=1e-3  SetiL0=off  InitialCurrent=0  Capacitance=Cfilter  Setx0=off  InitialVoltage=0  Measurements=None
  1 : PMIOPort  Side=Left
  2 : PMIOPort  Port=2  Side=Left
  tag scope: Ifilter_B=global
  wires:
  Current Measurement6/1 -> [Ifilter_B]
  connections:
  Current Measurement6/RConn1 -- Parallel RLC Branch/LConn1
  Parallel RLC Branch/RConn1 -- 2/RConn1
  1/RConn1 -- Breaker/LConn1
  Breaker/RConn1 -- Current Measurement6/LConn1

== system untitled/Filter2 ==
  Breaker : spsBreakerLib/Breaker  InitialState=1  SwitchingTimes=Topen_Filter  External=off  BreakerResistance=0.001  SnubberResistance=1e6  SnubberCapacitance=inf  Measurements=None  MoreParameters=on  NoBreakLoop=off
      settings: SourceProductBaseCode=PS
  Current Measurement6 : spsCurrentMeasurementLib/Current Measurement  PhasorSimulation=off  OutputType=Complex  PSBequivalent=0
  Parallel RLC Branch : spsParallelRLCBranchLib/Parallel RLC Branch  LConnTagsString=a  RConnTagsString=__new0  BranchType=RC  Resistance=Rfilter  Inductance=1e-3  SetiL0=off  InitialCurrent=0  Capacitance=Cfilter  Setx0=off  InitialVoltage=0  Measurements=None
  1 : PMIOPort  Side=Left
  2 : PMIOPort  Port=2  Side=Left
  tag scope: Ifilter_C=global
  wires:
  Current Measurement6/1 -> [Ifilter_C]
  connections:
  Parallel RLC Branch/RConn1 -- 2/RConn1
  Current Measurement6/RConn1 -- Parallel RLC Branch/LConn1
  Current Measurement6/LConn1 -- Breaker/RConn1
  1/RConn1 -- Breaker/LConn1

== system untitled/Filter3 ==
  Breaker : spsBreakerLib/Breaker  InitialState=1  SwitchingTimes=Topen_Filter  External=off  BreakerResistance=0.001  SnubberResistance=1e6  SnubberCapacitance=inf  Measurements=None  MoreParameters=on  NoBreakLoop=off
      settings: SourceProductBaseCode=PS
  Current Measurement6 : spsCurrentMeasurementLib/Current Measurement  PhasorSimulation=off  OutputType=Complex  PSBequivalent=0
  Parallel RLC Branch : spsParallelRLCBranchLib/Parallel RLC Branch  LConnTagsString=a  RConnTagsString=__new0  BranchType=RC  Resistance=Rfilter  Inductance=1e-3  SetiL0=off  InitialCurrent=0  Capacitance=Cfilter  Setx0=off  InitialVoltage=0  Measurements=None
  1 : PMIOPort  Side=Left
  2 : PMIOPort  Port=2  Side=Left
  tag scope: Ifilter_A1=global
  wires:
  Current Measurement6/1 -> [Ifilter_A1]
  connections:
  Parallel RLC Branch/RConn1 -- 2/RConn1
  Current Measurement6/RConn1 -- Parallel RLC Branch/LConn1
  1/RConn1 -- Breaker/LConn1
  Breaker/RConn1 -- Current Measurement6/LConn1

== system untitled/Filter4 ==
  Breaker : spsBreakerLib/Breaker  InitialState=1  SwitchingTimes=Topen_Filter  External=off  BreakerResistance=0.001  SnubberResistance=1e6  SnubberCapacitance=inf  Measurements=None  MoreParameters=on  NoBreakLoop=off
      settings: SourceProductBaseCode=PS
  Current Measurement6 : spsCurrentMeasurementLib/Current Measurement  PhasorSimulation=off  OutputType=Complex  PSBequivalent=0
  Parallel RLC Branch : spsParallelRLCBranchLib/Parallel RLC Branch  LConnTagsString=a  RConnTagsString=__new0  BranchType=RC  Resistance=Rfilter  Inductance=1e-3  SetiL0=off  InitialCurrent=0  Capacitance=Cfilter  Setx0=off  InitialVoltage=0  Measurements=None
  1 : PMIOPort  Side=Left
  2 : PMIOPort  Port=2  Side=Left
  tag scope: Ifilter_B1=global
  wires:
  Current Measurement6/1 -> [Ifilter_B1]
  connections:
  Current Measurement6/RConn1 -- Parallel RLC Branch/LConn1
  Parallel RLC Branch/RConn1 -- 2/RConn1
  1/RConn1 -- Breaker/LConn1
  Breaker/RConn1 -- Current Measurement6/LConn1

== system untitled/Filter5 ==
  Breaker : spsBreakerLib/Breaker  InitialState=1  SwitchingTimes=Topen_Filter  External=off  BreakerResistance=0.001  SnubberResistance=1e6  SnubberCapacitance=inf  Measurements=None  MoreParameters=on  NoBreakLoop=off
      settings: SourceProductBaseCode=PS
  Current Measurement6 : spsCurrentMeasurementLib/Current Measurement  PhasorSimulation=off  OutputType=Complex  PSBequivalent=0
  Parallel RLC Branch : spsParallelRLCBranchLib/Parallel RLC Branch  LConnTagsString=a  RConnTagsString=__new0  BranchType=RC  Resistance=Rfilter  Inductance=1e-3  SetiL0=off  InitialCurrent=0  Capacitance=Cfilter  Setx0=off  InitialVoltage=0  Measurements=None
  1 : PMIOPort  Side=Left
  2 : PMIOPort  Port=2  Side=Left
  tag scope: Ifilter_C1=global
  wires:
  Current Measurement6/1 -> [Ifilter_C1]
  connections:
  Parallel RLC Branch/RConn1 -- 2/RConn1
  Current Measurement6/RConn1 -- Parallel RLC Branch/LConn1
  Current Measurement6/LConn1 -- Breaker/RConn1
  1/RConn1 -- Breaker/LConn1

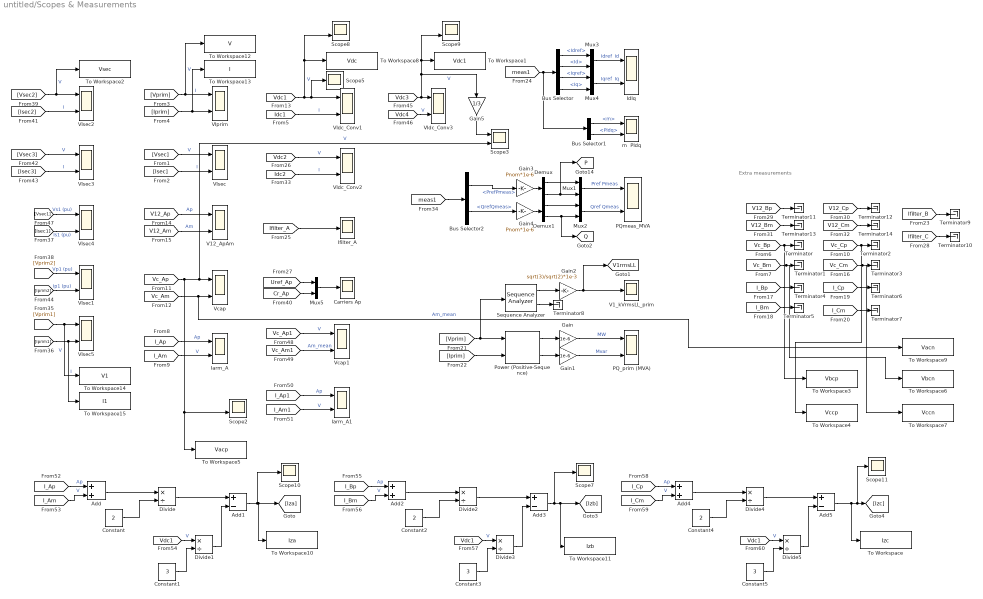
== system untitled/Scopes & Measurements ==
  note: Extra measurements
  Add : Sum
  Add1 : Sum  Inputs=+-
  Add2 : Sum
  Add3 : Sum  Inputs=+-
  Add4 : Sum
  Add5 : Sum  Inputs=+-
  Bus Selector : BusSelector  OutputSignals=Idref,Id,Iqref,Iq
  Bus Selector1 : BusSelector  OutputSignals=m,PIdq
  Bus Selector2 : BusSelector  OutputSignals=PrefPmeas,QrefQmeas
  Carriers Ap : Scope
  Constant : Constant  Value=2  SampleTime=-1
  Constant1 : Constant  Value=3  SampleTime=-1
  Constant2 : Constant  Value=2  SampleTime=-1
  Constant3 : Constant  Value=3  SampleTime=-1
  Constant4 : Constant  Value=2  SampleTime=-1
  Constant5 : Constant  Value=3  SampleTime=-1
  Demux : Demux  Outputs=2
  Demux1 : Demux  Outputs=2
  Divide{,1..5} (6 alike) : Product  Inputs=*/
  Gain : Gain  Gain=1e-6
  Gain1 : Gain  Gain=1e-6
  Gain2 : Gain  Gain=sqrt(3)/sqrt(2)*1e-3
  Gain3 : Gain  Gain=Pnom*1e-6
  Gain4 : Gain  Gain=Pnom*1e-6
  Gain5 : Gain  Gain=1/3
  Iarm_A : Scope  NumInputPorts=2
  Iarm_A1 : Scope  NumInputPorts=2
  IdIq : Scope  NumInputPorts=2
  Ifilter_A : Scope
  Mux{1..5} (5 alike) : Mux  Inputs=2
  PQ_prim (MVA) : Scope  NumInputPorts=2
  PQmeas_MVA : Scope  NumInputPorts=2
  Power (Positive-Sequence) : spsPowerPositiveSequenceLib/Power (Positive-Sequence)  Freq=Fnom  Vinit=[0, 0]  Iinit=[0, 0]  Ts=Ts_Power
      settings: SourceProductBaseCode=PS
  Scope{5,7,10..11} (4 alike) : Scope
  Scope{2..3,8..9} (4 alike) : Scope  NumInputPorts=2
  Sequence Analyzer : spsSequenceAnalyzerLib/Sequence Analyzer  Freq=Fnom  n=1  seq=Positive  InInit=[1, 0]  Ts=Ts_Power
      settings: SourceProductBaseCode=PS
  Terminator{,1..14} (15 alike) : Terminator
  To Workspace : ToWorkspace  VariableName=Izc  SaveFormat=Timeseries  SampleTime=-1
  To Workspace1 : ToWorkspace  VariableName=Vdc1  SaveFormat=Timeseries  SampleTime=-1
  To Workspace10 : ToWorkspace  VariableName=Iza  SaveFormat=Timeseries  SampleTime=-1
  To Workspace11 : ToWorkspace  VariableName=Izb  SaveFormat=Timeseries  SampleTime=-1
  To Workspace12 : ToWorkspace  VariableName=V  SaveFormat=Timeseries  SampleTime=-1
  To Workspace13 : ToWorkspace  VariableName=I  SaveFormat=Timeseries  SampleTime=-1
  To Workspace14 : ToWorkspace  VariableName=V1  SaveFormat=Timeseries  SampleTime=-1
  To Workspace15 : ToWorkspace  VariableName=I1  SaveFormat=Timeseries  SampleTime=-1
  To Workspace2 : ToWorkspace  VariableName=Vsec  SaveFormat=Timeseries  SampleTime=-1
  To Workspace3 : ToWorkspace  VariableName=Vbcp  SaveFormat=Timeseries  SampleTime=-1
  To Workspace4 : ToWorkspace  VariableName=Vccp  SaveFormat=Timeseries  SampleTime=-1
  To Workspace5 : ToWorkspace  VariableName=Vacp  SaveFormat=Timeseries  SampleTime=-1
  To Workspace6 : ToWorkspace  VariableName=Vbcn  SaveFormat=Timeseries  SampleTime=-1
  To Workspace7 : ToWorkspace  VariableName=Vccn  SaveFormat=Timeseries  SampleTime=-1
  To Workspace8 : ToWorkspace  VariableName=Vdc  SaveFormat=Timeseries  SampleTime=-1
  To Workspace9 : ToWorkspace  VariableName=Vacn  SaveFormat=Timeseries  SampleTime=-1
  V12_ApAm : Scope  NumInputPorts=2
  V1_kVrmsLL_prim : Scope
  VIdc_Conv1 : Scope  NumInputPorts=2
  VIdc_Conv2 : Scope  NumInputPorts=2
  VIdc_Conv3 : Scope  NumInputPorts=2
  VIprim : Scope  NumInputPorts=2
  VIsec{,1..5} (6 alike) : Scope  NumInputPorts=2
  Vcap : Scope  NumInputPorts=2
  Vcap1 : Scope  NumInputPorts=2
  m  PIdq : Scope  NumInputPorts=2
  tag scope: P=global, Q=global, V1rmsLL=global
  wires:
  Mux5/1 -> Carriers Ap/1
  [Cr_Ap] -> Mux5/2
  [Uref_Ap] -> Mux5/1
  [Vc_Am] -> To Workspace9/1, Vcap/2  "Am_mean"
  [Idc2] -> VIdc_Conv2/2  "I"
  [Vdc2] -> VIdc_Conv2/1  "V"
  Gain4/1 -> Demux1/1
  Gain3/1 -> Demux/1
  Mux2/1 -> PQmeas_MVA/2  "Qref Qmeas"
  Bus Selector2/2 -> Gain4/1  "<QrefQmeas>"
  Bus Selector2/1 -> Gain3/1  "<PrefPmeas>"
  Mux1/1 -> PQmeas_MVA/1  "Pref Pmeas"
  [meas1] -> Bus Selector2/1
  Gain2/1 -> V1_kVrmsLL_prim/1, [V1rmsLL]
  Gain1/1 -> PQ_prim (MVA)/2  "Mvar"
  Gain/1 -> PQ_prim (MVA)/1  "MW"
  [V12_Cm] -> Terminator14/1
  [V12_Bm] -> Terminator13/1
  [V12_Cp] -> Terminator12/1
  [V12_Bp] -> Terminator11/1
  [Ifilter_C] -> Terminator10/1
  [Ifilter_B] -> Terminator9/1
  Sequence Analyzer/1 -> Gain2/1
  Power (Positive-Sequence)/2 -> Gain1/1
  Power (Positive-Sequence)/1 -> Gain/1
  Sequence Analyzer/2 -> Terminator8/1
  [Iprim] -> Power (Positive-Sequence)/2
  [Vprim] -> Power (Positive-Sequence)/1, Sequence Analyzer/1
  [Idc1] -> VIdc_Conv1/2  "I"
  [Vdc1] -> Scope8/2, To Workspace8/1, Scope5/1, VIdc_Conv1/1  "V"
  [Ifilter_A] -> Ifilter_A/1
  Bus Selector/4 -> Mux4/2  "<Iq>"
  Bus Selector/3 -> Mux4/1  "<Iqref>"
  Bus Selector/2 -> Mux3/2  "<Id>"
  Bus Selector/1 -> Mux3/1  "<Idref>"
  Mux4/1 -> IdIq/2  "Iqref  Iq"
  Mux3/1 -> IdIq/1  "Idref  Id"
  Bus Selector1/2 -> m  PIdq/2  "<PIdq>"
  Bus Selector1/1 -> m  PIdq/1  "<m>"
  [meas1] -> Bus Selector/1, Bus Selector1/1
  [I_Cm] -> Terminator7/1
  [I_Cp] -> Terminator6/1
  [I_Bm] -> Terminator5/1
  [I_Bp] -> Terminator4/1
  [I_Ap] -> Iarm_A/1  "Ap"
  [Vc_Cm] -> To Workspace7/1, Terminator3/1
  [Vc_Cp] -> To Workspace4/1, Terminator2/1
  [Vc_Bm] -> To Workspace6/1, Terminator1/1
  [Vc_Bp] -> To Workspace3/1, Terminator/1
  [V12_Am] -> V12_ApAm/2  "Am"
  [V12_Ap] -> V12_ApAm/1  "Ap"
  [Vsec] -> VIsec/1  "V"
  [Isec] -> VIsec/2  "I"
  [Vprim] -> To Workspace12/1, VIprim/1  "V"
  [Iprim] -> To Workspace13/1, VIprim/2  "I"
  Demux/1 -> Mux1/1
  Demux/2 -> [P], Mux1/2
  Demux1/1 -> Mux2/1
  Demux1/2 -> [Q], Mux2/2
  [Vsec3] -> VIsec3/1  "V"
  [Isec3] -> VIsec3/2  "I"
  [Isec2] -> VIsec2/2  "I"
  [Vsec2] -> To Workspace2/1, VIsec2/1  "V"
  [Iprim2] -> VIsec1/2  "Ip1 (pu)"
  [Isec1] -> VIsec4/2  "Is1 (pu)"
  [Vprim2] -> VIsec1/1  "Vp1 (pu)"
  [Vsec1] -> VIsec4/1  "Vs1 (pu)"
  [Vdc3] -> Gain5/1, Scope9/2, To Workspace1/1, VIdc_Conv3/1  "V"
  [Vdc4] -> VIdc_Conv3/2  "V"
  [I_Ap1] -> Iarm_A1/1  "Ap"
  [Vc_Am1] -> Vcap1/2  "Am_mean"
  [Vc_Ap] -> To Workspace5/1, Scope2/2, Scope3/2, Vcap/1  "V"
  [I_Am] -> Iarm_A/2  "V"
  [Vc_Ap1] -> Vcap1/1  "V"
  [I_Am1] -> Iarm_A1/2  "V"
  ? -> Scope2/1
  Gain5/1 -> Scope3/1
  ? -> Scope8/1
  ? -> Scope9/1
  [Vprim1] -> To Workspace14/1, VIsec5/1  "V"
  [Iprim1] -> To Workspace15/1, VIsec5/2  "I"
  [I_Ap] -> Add/1  "Ap"
  [I_Am] -> Add/2  "V"
  Add/1 -> Divide/1
  Constant/1 -> Divide/2
  Divide/1 -> Add1/1
  Divide1/1 -> Add1/2
  [Vdc1] -> Divide1/1  "V"
  Constant1/1 -> Divide1/2
  Add1/1 -> Scope10/1, To Workspace10/1, [Iza]
  [Vdc1] -> Divide3/1  "V"
  [I_Bm] -> Add2/2  "V"
  Add2/1 -> Divide2/1
  Constant3/1 -> Divide3/2
  Divide3/1 -> Add3/2
  [I_Bp] -> Add2/1  "Ap"
  Constant2/1 -> Divide2/2
  Divide2/1 -> Add3/1
  Add3/1 -> Scope7/1, To Workspace11/1, [Izb]
  [Vdc1] -> Divide5/1  "V"
  [I_Cm] -> Add4/2  "V"
  Add4/1 -> Divide4/1
  Constant5/1 -> Divide5/2
  Divide5/1 -> Add5/2
  [I_Cp] -> Add4/1  "Ap"
  Constant4/1 -> Divide4/2
  Divide4/1 -> Add5/1
  Add5/1 -> To Workspace/1, Scope11/1, [Izc]

== system untitled/SubSystem ==

== system untitled/Subsystem ==
  Current Measurement1 : spsCurrentMeasurementLib/Current Measurement  PhasorSimulation=off  OutputType=Complex  PSBequivalent=0
  Voltage Measurement : spsVoltageMeasurementLib/Voltage Measurement  PhasorSimulation=off  OutputType=Complex  PSBequivalent=0
  I1 : PMIOPort  Side=Left
  I2 : PMIOPort  Port=2  Side=Left
  O1 : PMIOPort  Port=3  Side=Right
  O2 : PMIOPort  Port=4  Side=Right
  tag scope: I_Ap=global, V12_Ap=global
  wires:
  Current Measurement1/1 -> [I_Ap]
  Voltage Measurement/1 -> [V12_Ap]
  connections:
  Current Measurement1/RConn1 -- Voltage Measurement/LConn1 -- I1/RConn1
  Current Measurement1/LConn1 -- O1/RConn1
  I2/RConn1 -- Voltage Measurement/LConn2 -- O2/RConn1

== system untitled/Subsystem1 ==
  Current Measurement1 : spsCurrentMeasurementLib/Current Measurement  PhasorSimulation=off  OutputType=Complex  PSBequivalent=0
  Voltage Measurement : spsVoltageMeasurementLib/Voltage Measurement  PhasorSimulation=off  OutputType=Complex  PSBequivalent=0
  I1 : PMIOPort  Side=Left
  I2 : PMIOPort  Port=2  Side=Left
  O1 : PMIOPort  Port=3  Side=Right
  O2 : PMIOPort  Port=4  Side=Right
  tag scope: I_Am=global, V12_Am=global
  wires:
  Voltage Measurement/1 -> [V12_Am]
  Current Measurement1/1 -> [I_Am]
  connections:
  Voltage Measurement/LConn2 -- O2/RConn1 -- I2/RConn1
  Current Measurement1/LConn1 -- O1/RConn1
  Voltage Measurement/LConn1 -- Current Measurement1/RConn1 -- I1/RConn1

== system untitled/Subsystem10 ==
  Current Measurement1 : spsCurrentMeasurementLib/Current Measurement  PhasorSimulation=off  OutputType=Complex  PSBequivalent=0
  Voltage Measurement : spsVoltageMeasurementLib/Voltage Measurement  PhasorSimulation=off  OutputType=Complex  PSBequivalent=0
  I1 : PMIOPort  Side=Left
  I2 : PMIOPort  Port=2  Side=Left
  O1 : PMIOPort  Port=3  Side=Right
  O2 : PMIOPort  Port=4  Side=Right
  tag scope: I_Cp1=global, V12_Cp1=global
  wires:
  Current Measurement1/1 -> [I_Cp1]
  Voltage Measurement/1 -> [V12_Cp1]
  connections:
  I1/RConn1 -- Current Measurement1/RConn1 -- Voltage Measurement/LConn1
  Current Measurement1/LConn1 -- O1/RConn1
  I2/RConn1 -- O2/RConn1 -- Voltage Measurement/LConn2
